simulink model "EKMSL"  (R2020b)
settings: Solver=VariableStepAuto  StartTime=0.0  StopTime=10.0  MaxStep=EKM.T_ABS/25  RelTol=1e-4
undefined symbols (not defined in the file or in its folder): EKM
libraries: simulink x1
settings Model: Creator=Szalay  LastModifiedBy=Szalay

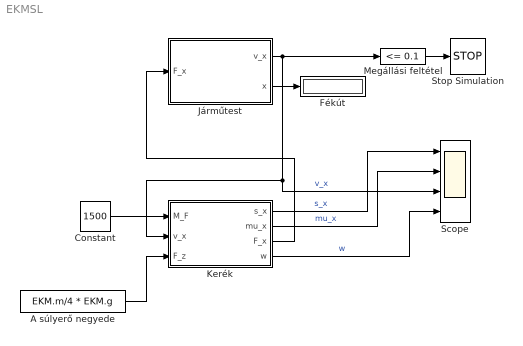
== system EKMSL ==
  A súlyerő negyede : Constant  Value=EKM.m/4 * EKM.g
  Constant : Constant  Value=1500
  Fékút : Display
  Járműtest : Subsystem  mask(Járműtest){m=EKM.m, c_W=EKM.c_W, rho_L=EKM.rho_L, A_0=EKM.A_0, v_0=EKM.v_0, x_0=0}
      mask prompts: m "Tömeg [kg]"; c_W "Légellenállási tényező"; rho_L "A levegő sűrűsége [kg/m^3]"; A_0 "Homlokfelület [m^2]"; v_0 "Kezdeti sebesség [m/s]"; x_0 "Kezdeti hely [m]"
      mask help: A járműtest hosszirányú mozgásegyenlete.
      mask DialogControl ParameterGroupVar Prompt: A járműtest tömege
      mask DialogControl Container3 Prompt: Légellenállás
      mask DialogControl Container4 Prompt: Kezdeti értékek
      mask Display:
      | text(0.5, 0.5, '{\bfJárműtest}', ...
      | 	'HorizontalAlignment', 'center', ...
      | 	'texmode', 'on' ...
      | 	);
      | 
      | port_label('input', 1, '{\itF_x}', 'texmode', 'on');
      | 
      | port_label('output', 1, '{\itv_x}', 'texmode', 'on');
      | port_label('output', 2, '{\itx}', 'texmode', 'on');
  Kerék : Subsystem  mask(Kerékmodell){R=EKM.R_K, J=EKM.J_K, B=EKM.B_H, w_0=EKM.w_0}
      mask prompts: R "Keréksugár [m]"; J "Tehetetlenségi nyomaték [kg m^2]"; B "Forgási súrlódási tényező [N m/(rad/s)]"; w_0 "Kezdeti keréksebesség [rad/s]"
      mask help: A kerékmodell a Pacejka-féle gumiabroncs modellel és féknyomaték-korlátozással.
      mask DialogControl WheelParameters Prompt: Kerékjellemzők
      mask DialogControl DriveTrain Prompt: A hajtáslánc jellemzői
      mask DialogControl InitialValues Prompt: Kezdeti értékek
      mask Display:
      | text(0.5, 0.5, '{\bfKerék}', ...
      | 	'HorizontalAlignment', 'center', ...
      | 	'texmode', 'on' ...
      | 	);
      | 
      | port_label('input', 1, '{\itM_F}', 'texmode', 'on');
      | port_label('input', 2, '{\itv_x}', 'texmode', 'on');
      | port_label('input', 3, '{\itF_z}', 'texmode', 'on');
      | 
      | port_label('output', 1, '{\its_x}', 'texmode', 'on');
      | port_label('output', 2, '{\it\mu_x}', 'texmode', 'on');
      | port_label('output', 3, '{\itF_x}', 'texmode', 'on');
      | port_label('output', 4, '{\it\omega}', 'texmode', 'on');
  Megállási feltétel : simulink/Logic and Bit Operations/Compare To Constant  relop=<=  const=0.1  OutDataTypeStr=boolean
  Scope : Scope  NumInputPorts=4
  Stop Simulation : Stop
  wires:
  Kerék/3(F_x) -> Járműtest/1(F_x)
  Járműtest/1(v_x) -> Megállási feltétel/1, Scope/3, Kerék/2(v_x)  "v_x"
  Járműtest/2(x) -> Fékút/1
  Megállási feltétel/1 -> Stop Simulation/1
  Kerék/1(s_x) -> Scope/1  "s_x"
  Kerék/2(mu_x) -> Scope/2  "mu_x"
  Kerék/4(w) -> Scope/4  "w"
  A súlyerő negyede/1 -> Kerék/3(F_z)
  Constant/1 -> Kerék/1(M_F)

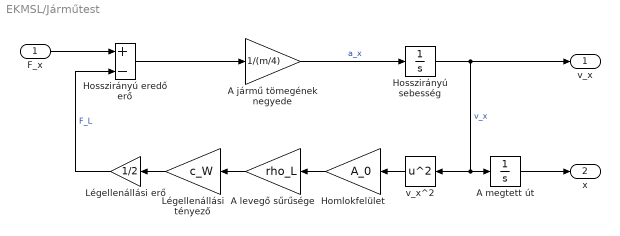
== system EKMSL/Járműtest ==
  F_x : Inport
  A jármű tömegének negyede : Gain  Gain=1/(m/4)
  A levegő sűrűsége : Gain  Gain=rho_L
  A megtett út : Integrator  InitialCondition=x_0
  Homlokfelület : Gain  Gain=A_0
  Hosszirányú sebesség : Integrator  InitialCondition=v_0
  Hosszirányú eredő erő : Sum  Inputs=+-
  Légellenállási erő : Gain  Gain=1/2
  Légellenállási tényező : Gain  Gain=c_W
  v_x^2 : Math  Operator=square  SaturateOnIntegerOverflow=on
  v_x : Outport
  x : Outport  Port=2
  wires:
  Homlokfelület/1 -> A levegő sűrűsége/1
  v_x^2/1 -> Homlokfelület/1
  Légellenállási erő/1 -> Hosszirányú eredő erő/2  "F_L"
  F_x/1 -> Hosszirányú eredő erő/1
  Légellenállási tényező/1 -> Légellenállási erő/1
  Hosszirányú sebesség/1 -> v_x/1, A megtett út/1, v_x^2/1  "v_x"
  Hosszirányú eredő erő/1 -> A jármű tömegének negyede/1
  A levegő sűrűsége/1 -> Légellenállási tényező/1
  A jármű tömegének negyede/1 -> Hosszirányú sebesség/1  "a_x"
  A megtett út/1 -> x/1

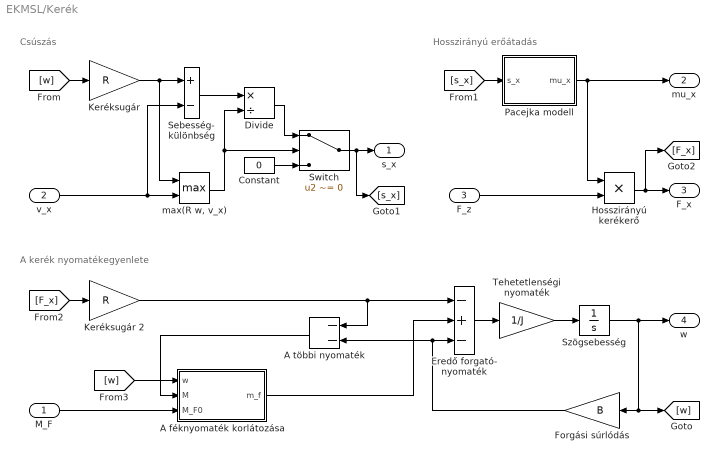
== system EKMSL/Kerék ==
  note: A kerék nyomatékegyenlete
  note: Hosszirányú erőátadás
  note: Csúszás
  M_F : Inport
  v_x : Inport  Port=2
  F_z : Inport  Port=3
  A féknyomaték korlátozása : MATLAB Function  TreatAsAtomicUnit=on
  A többi nyomaték : Sum  Inputs=--
  Constant : Constant  Value=0
  Divide : Product  Inputs=*/
  Eredő forgató- nyomaték : Sum  Inputs=-+-
  Forgási súrlódás : Gain  Gain=B
  Hosszirányú kerékerő : Product
  Keréksugár : Gain  Gain=R
  Keréksugár 2 : Gain  Gain=R
  Pacejka modell : MATLAB Function  TreatAsAtomicUnit=on
  Sebesség- különbség : Sum  Inputs=+-
  Switch : Switch  Criteria=u2 ~= 0
  Szögsebesség : Integrator  InitialCondition=w_0  LimitOutput=on  LowerSaturationLimit=0
  Tehetetlenségi nyomaték : Gain  Gain=1/J
  "max(R w, v_x)" : MinMax  Function=max  Inputs=2
  s_x : Outport
  mu_x : Outport  Port=2
  F_x : Outport  Port=3
  w : Outport  Port=4
  wires:
  Szögsebesség/1 -> w/1, [w], Forgási súrlódás/1
  [w] -> Keréksugár/1
  Keréksugár/1 -> "max(R w, v_x)"/1, Sebesség- különbség/1
  v_x/1 -> "max(R w, v_x)"/2, Sebesség- különbség/2
  Sebesség- különbség/1 -> Divide/1
  "max(R w, v_x)"/1 -> Switch/2, Divide/2
  Divide/1 -> Switch/1
  Constant/1 -> Switch/3
  Switch/1 -> [s_x], s_x/1
  [s_x] -> Pacejka modell/1(s_x)
  Pacejka modell/1(mu_x) -> Hosszirányú kerékerő/1, mu_x/1
  F_z/1 -> Hosszirányú kerékerő/2
  Hosszirányú kerékerő/1 -> [F_x], F_x/1
  Tehetetlenségi nyomaték/1 -> Szögsebesség/1
  Eredő forgató- nyomaték/1 -> Tehetetlenségi nyomaték/1
  Forgási súrlódás/1 -> Eredő forgató- nyomaték/3, A többi nyomaték/2
  [F_x] -> Keréksugár 2/1
  Keréksugár 2/1 -> A többi nyomaték/1, Eredő forgató- nyomaték/1
  M_F/1 -> A féknyomaték korlátozása/3(M_F0)
  A féknyomaték korlátozása/1(m_f) -> Eredő forgató- nyomaték/2
  [w] -> A féknyomaték korlátozása/1(w)
  A többi nyomaték/1 -> A féknyomaték korlátozása/2(M)

== matlab function EKMSL/Kerék/Pacejka modell ==
  data: s_x input; mu_x output
function mu_x = Pacejka(s_x)

mu_x = EKM.PacejkaLongitudinalForceCoefficient(s_x);

== matlab function EKMSL/Kerék/A féknyomaték korlátozása ==
  data: w input; m_f output; M input; M_F0 input
function m_f = M_F(w, M, M_F0)

m_f = EKM.M_F(w, M, M_F0);
